simulink model "px4demo_ParameterUpdate_CSC_example"  (R2017b)
settings: Solver=FixedStepAuto  StartTime=0.0  StopTime=inf  RelTol=1e-3  EnableMultiTasking=on
InitFcn:
  | CAL_GYRO0_XSCALE = Pixhawk_CSC.Parameter( {single(1), 'CAL_GYRO0_XSCALE'}  )
  | CAL_GYRO0_YSCALE = Pixhawk_CSC.Parameter( {single(1), 'CAL_GYRO0_YSCALE'}  )
  | CAL_GYRO0_ZSCALE = Pixhawk_CSC.Parameter( {single(1), 'CAL_GYRO0_ZSCALE'}  )
  | 
  | CAL_GYRO0_XOFF = Pixhawk_CSC.Parameter( {single(0), 'CAL_GYRO0_XOFF'} )
  | CAL_GYRO0_YOFF = Pixhawk_CSC.Parameter( {single(0), 'CAL_GYRO0_YOFF'} )
  | CAL_GYRO0_ZOFF = Pixhawk_CSC.Parameter( {single(0), 'CAL_GYRO0_ZOFF'} )
libraries: pixhawk_slib_misc_utils x1
Description:
  | PX4 PSP Demo Model - Paramater Update Custom Storage Classes
  | 
  | The Pixhawk Px4FMUv2 uses many parameters to store and access during various operations.
  | 
  | Much of these include sensor/actuator calibration data and are stored in flash memory which is accessible by MTD via NuttX.
  | 
  | You can read the default parameters or follow the guide to creating your own parameters.
  | 
  | The Pixhawk PSP allows you to access these parameters using Embedded Coder's Custom Storage Class feature.
  | 
  | A parameter is first defined in the MATLAB workspace with specific parameter properties which is then accessed in the generated code.
  | 
  | To make use of this, use the following syntax:
  | 
  | Pixhawk_CSC.Parameter( CELL_ARRAY )
  | 
  | Where CELL_ARRAY is a MATLAB cell array composed of a value (int32 or single) and a string of the parameter. For instance:
  | 
  | CAL_GYRO0_XSCALE = Pixhawk_CSC.Parameter( {single(1), 'CAL_GYRO0_XSCALE'}  )
  | 
  | Parameters can either be int32 or single/floating precision. Please ensure you select the correct data type and the the string name matches.
  | 
  | Note that for the model below, all parameters have been defined in the model's InitFcn callback function
  | 
  | The ParamUpdate block on the left provides a mechanism to update the parameters using QGroundControl. A uORB topic is subscribed to "parameter_update" to check to see when parameters received an update. You can ues the block UI to specify which parameters to update in the list.
settings Model: SimulationMode=external  Creator=darenlee  LastModifiedBy=skuznick
settings SolverCC: PositivePriorityOrder=on
settings DataIOCC: LimitDataPoints=on
settings OptimizationCC: DefaultParameterBehavior=Inlined  LifeSpan=1  MaxStackSize=64
settings DebuggingCC: AllowSymbolicDim=off  SFUnexpectedBacktrackingDiag=warning  SFNoUnconditionalDefaultTransitionDiag=warning  SFExecutionAtInitializationDiag=none
settings HardwareCC: ProdBitPerPointer=32  ProdBitPerSizeT=32  ProdBitPerPtrDiffT=32  ProdLargestAtomicInteger=Long  ProdLargestAtomicFloat=Double  ProdWordSize=32  ProdHWDeviceType=ARM Compatible->ARM Cortex
settings ModelReferenceCC: PropagateSignalLabelsOutOfModel=off
settings SFSimCC: MATLABDynamicMemAlloc=off
settings RTWCC: SystemTargetFile=ert.tlc  HardwareBoard=Pixhawk PX4  TemplateMakefile=ert_default_tmf  GenerateReport=on  Toolchain=Pixhawk Toolchain  IncludeHyperlinkInReport=on  LaunchReport=on  GenerateTraceInfo=on  GenerateTraceReport=on  GenerateTraceReportSl=on  GenerateTraceReportSf=on  GenerateTraceReportEml=on
settings RTWCC: CustomHeaderCode=|
  | #include <px4_config.h>
  | #include <px4_tasks.h>
  | #include <px4_posix.h>
  | #include <unistd.h>
  | #include <stdio.h>
  | #include <poll.h>
  | #include <string.h>
settings CodeAppCC: ForceParamTrailComments=on  IgnoreCustomStorageClasses=off  OperatorAnnotations=on  StateflowObjectComments=on  MATLABSourceComments=on
settings ERTTargetCC: MultiwordLength=2048  ExtModeTransport=1  ExtModeMexFile=ext_serial_win32_comm  ExtModeMexArgs=1 7 115200  InlinedParameterPlacement=NonHierarchical  ERTCustomFileTemplate=px4_codertarget_file_process.tlc  ConvertIfToSwitch=off  SuppressUnreachableDefaultCases=off
settings ConfigComp: CovMetricSettings=dw  CovHtmlReporting=on  CovSaveCumulativeToWorkspaceVar=on  CovSaveSingleToWorkspaceVar=on  CovExternalEMLEnable=off

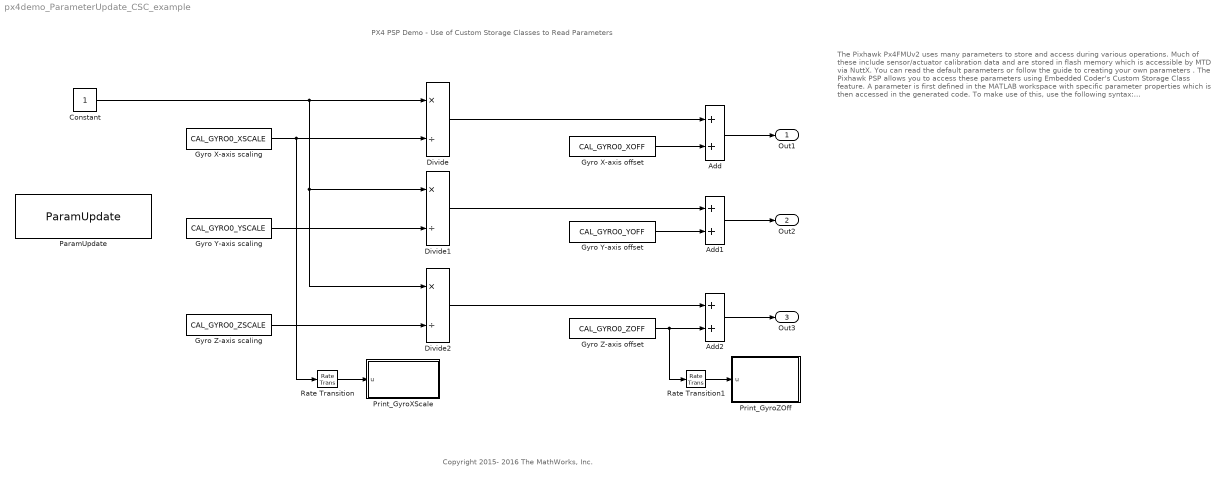
== system px4demo_ParameterUpdate_CSC_example ==
  note: PX4 PSP Demo - Use of Custom Storage Classes to Read Parameters
  note: The Pixhawk Px4FMUv2 uses many parameters to store and access during various operations.
      |
      | Much of these include sensor/actuator calibration data and are stored in flash memory which is accessible by MTD via NuttX.
      |
      | You can read the default parameters or follow the guide to creating your own parameters .
      |
      | The Pixhawk PSP allows you to access these parameters using Embedded Coder's Custom Storage Class feature.
      |
      | A parameter is first defined in the MATLAB workspace with specific parameter properties which is then accessed in the generated code.
      |
      | To make use of this, use the following syntax:
      |
      | Pixhawk_CSC.Parameter( CELL_ARRAY )
      |
      | Where CELL_ARRAY is a MATLAB cell array composed of a value (int32 or single) and a string of the parameter. For instance:
      |
      | CAL_GYRO0_XSCALE = Pixhawk_CSC.Parameter( {single(1), 'CAL_GYRO0_XSCALE'} )
      |
      | Parameters can either be int32 or single/floating precision. Please ensure you select the correct data type and the the string name matches.
      |
      | Note that for the model below, all parameters have been defined in the model's InitFcn callback function
      |
      | The ParamUpdate block on the left provides a mechanism to update the parameters using QGroundControl. A uORB topic is subscribed to "parameter_update" to check to see when parameters received an update. You can ues the block UI to specify which parameters to update in the list.
  note: Copyright 2015- 2016 The MathWorks, Inc.
  Add : Sum
  Add1 : Sum
  Add2 : Sum
  Constant : Constant  OutDataTypeStr=single  SampleTime=1/10
  Divide : Product  Inputs=*/
  Divide1 : Product  Inputs=*/
  Divide2 : Product  Inputs=*/
  "Gyro X-axis offset\t" : Constant  Value=CAL_GYRO0_XOFF  SampleTime=-1
  Gyro X-axis scaling : Constant  Value=CAL_GYRO0_XSCALE  SampleTime=-1
  Gyro Y-axis offset : Constant  Value=CAL_GYRO0_YOFF  SampleTime=-1
  Gyro Y-axis scaling : Constant  Value=CAL_GYRO0_YSCALE  SampleTime=-1
  Gyro Z-axis offset : Constant  Value=CAL_GYRO0_ZOFF  SampleTime=-1
  Gyro Z-axis scaling : Constant  Value=CAL_GYRO0_ZSCALE  SampleTime=-1
  ParamUpdate : pixhawk_slib_misc_utils/ParamUpdate  Unformatted_StrSet=0  TLC_StrSet=0  NumParams=0  Ts=0
      settings: SourceProductName=Pixhawk Target Blocks
  Print_GyroXScale : MATLAB Function  TreatAsAtomicUnit=on
  Print_GyroZOff : MATLAB Function  TreatAsAtomicUnit=on
  Rate Transition : RateTransition  OutPortSampleTime=0.5
  Rate Transition1 : RateTransition  OutPortSampleTime=0.5
  Out1 : Outport
  Out2 : Outport  Port=2
  Out3 : Outport  Port=3
  wires:
  "Gyro X-axis offset\t"/1 -> Add/2
  Gyro Y-axis offset/1 -> Add1/2
  Constant/1 -> Divide2/1, Divide1/1, Divide/1
  Divide/1 -> Add/1
  Divide1/1 -> Add1/1
  Divide2/1 -> Add2/1
  Add/1 -> Out1/1
  Add1/1 -> Out2/1
  Add2/1 -> Out3/1
  Gyro Y-axis scaling/1 -> Divide1/2
  Gyro Z-axis scaling/1 -> Divide2/2
  Gyro X-axis scaling/1 -> Rate Transition/1, Divide/2
  Gyro Z-axis offset/1 -> Rate Transition1/1, Add2/2
  Rate Transition/1 -> Print_GyroXScale/1(u)
  Rate Transition1/1 -> Print_GyroZOff/1(u)

== matlab function px4demo_ParameterUpdate_CSC_example/Print_GyroZOff ==
  data: u input
function print_fcn(u)
if coder.target('rtw')
msg_str = coder.const(['CAL_GYRO0_ZOFF = %8.4f',uint8(10),uint8(0)]);
coder.ceval('PX4_INFO',coder.rref(msg_str),u);
end
end

== matlab function px4demo_ParameterUpdate_CSC_example/Print_GyroXScale ==
  data: u input
function print_fcn(u)
if coder.target('rtw')
msg_str = coder.const(['CAL_GYRO0_XSCALE = %8.4f',uint8(10),uint8(0)]);
coder.ceval('PX4_INFO',coder.rref(msg_str),u);
end
end
